simulink model "TorqueControlConfig"  (R2023b)
settings: Solver=VariableStepAuto  StartTime=0.0  StopTime=20  RelTol=1e-3
PostLoadFcn:
  | run('ParametricRobotLoader.m')
  | run('ParametricRobotParameters');
  | TsCtrl=0.005
  | Config.Mode=ones(1,6)
  | Config.Value = zeros(1,6)
undefined symbols (not defined in the file): ctrlLowerLimit, ctrlUpperLimit
libraries: nesl_utility x19, fl_lib x6, slpidlib x6, sm_lib x3, simulink x2, robotmaniplib x1
(part 1 of 2)
settings Model: PauseTimes=1  Creator=jjha  LastModifiedBy=abirdas
settings OptimizationCC: ReuseModelBlockBuffer=off
settings SimscapeCC: SimscapeLogType=all

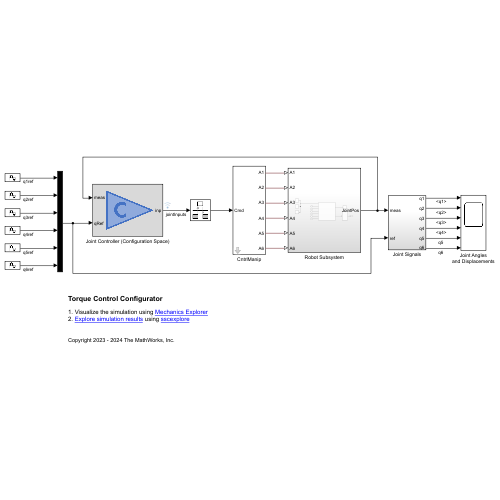
[thumbnail: Simulink's stored preview of the top-level diagram]
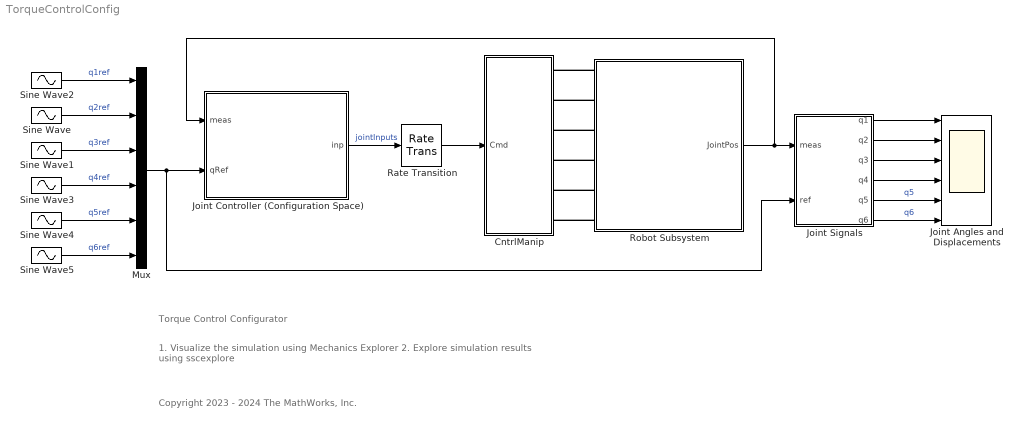
== system TorqueControlConfig ==
  note: Torque Control Configurator
  note: 1. Visualize the simulation using Mechanics Explorer
      | 2. Explore simulation results using sscexplore
  note: Copyright 2023 - 2024 The MathWorks, Inc.
  CntrlManip : Subsystem  mask{ControlSel=[1,1,1,1,1,1], ControlVal=Config.Value}
      mask prompts: ControlSel "Control Manipulator Selector"; ControlVal "Control Manipulator Value"
  Joint Angles and Displacements : Scope  NumInputPorts=6
  Joint Controller (Configuration Space) : Subsystem  VariantControl=ctrlType==1
      mask Display: image('Controller.PNG')
  Joint Signals : Subsystem
  Mux : Mux  Inputs=6
  Rate Transition : RateTransition
  Robot Subsystem : Subsystem
  Sine Wave : Sin  Amplitude=pi/4  Frequency=2  SampleTime=TsCtrl
  Sine Wave1 : Sin  Amplitude=pi/2  Frequency=1.5  SampleTime=TsCtrl
  Sine Wave2 : Sin  Amplitude=2*pi/3  Frequency=0.4  SampleTime=TsCtrl
  Sine Wave3 : Sin  Amplitude=pi/3  SampleTime=TsCtrl
  Sine Wave4 : Sin  Amplitude=2  Frequency=0.5  SampleTime=TsCtrl
  Sine Wave5 : Sin  Amplitude=pi/3  Frequency=2  SampleTime=TsCtrl
  wires:
  Joint Signals/4(q4) -> Joint Angles and Displacements/4
  Joint Signals/2(q2) -> Joint Angles and Displacements/2
  Robot Subsystem/1(JointPos) -> Joint Controller (Configuration Space)/1(meas), Joint Signals/1(meas)
  Joint Signals/3(q3) -> Joint Angles and Displacements/3
  Joint Signals/1(q1) -> Joint Angles and Displacements/1
  Joint Controller (Configuration Space)/1(inp) -> Rate Transition/1  "jointInputs"
  Mux/1 -> Joint Signals/2(ref), Joint Controller (Configuration Space)/2(qRef)
  Joint Signals/5(q5) -> Joint Angles and Displacements/5  "q5"
  Joint Signals/6(q6) -> Joint Angles and Displacements/6  "q6"
  Sine Wave2/1 -> Mux/1  "q1ref"
  Sine Wave/1 -> Mux/2  "q2ref"
  Sine Wave1/1 -> Mux/3  "q3ref"
  Sine Wave3/1 -> Mux/4  "q4ref"
  Sine Wave4/1 -> Mux/5  "q5ref"
  Sine Wave5/1 -> Mux/6  "q6ref"
  Rate Transition/1 -> CntrlManip/1(Cmd)
  connections:
  Robot Subsystem/LConn1 -- CntrlManip/RConn1
  Robot Subsystem/LConn2 -- CntrlManip/RConn2
  Robot Subsystem/LConn3 -- CntrlManip/RConn3
  Robot Subsystem/LConn4 -- CntrlManip/RConn4
  Robot Subsystem/LConn5 -- CntrlManip/RConn5
  Robot Subsystem/LConn6 -- CntrlManip/RConn6

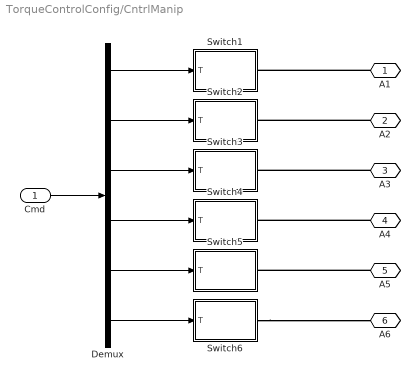
== system TorqueControlConfig/CntrlManip ==
  Cmd : Inport
  Demux : Demux  Outputs=6
  Switch1 : Subsystem  mask{ManipCtrl=ControlSel(1), ManipValue=ControlVal(1)}
      mask prompts: ManipCtrl "Control Selector"; ManipValue "Control Value"
      mask DialogControl Manipulator Prompt: Torque or Motion control
  Switch2 : Subsystem  mask{ManipCtrl=ControlSel(2), ManipValue=ControlVal(2)}
      mask prompts: ManipCtrl "Control Selector"; ManipValue "Control Value"
      mask DialogControl Manipulator Prompt: Torque or Motion control
  Switch3 : Subsystem  mask{ManipCtrl=ControlSel(3), ManipValue=ControlVal(3)}
      mask prompts: ManipCtrl "Control Selector"; ManipValue "Control Value"
      mask DialogControl Manipulator Prompt: Torque or Motion control
  Switch4 : Subsystem  mask{ManipCtrl=ControlSel(4), ManipValue=ControlVal(4)}
      mask prompts: ManipCtrl "Control Selector"; ManipValue "Control Value"
      mask DialogControl Manipulator Prompt: Torque or Motion control
  Switch5 : Subsystem  mask{ManipCtrl=ControlSel(5), ManipValue=ControlVal(5)}
      mask prompts: ManipCtrl "Control Selector"; ManipValue "Control Value"
      mask DialogControl Manipulator Prompt: Torque or Motion control
  Switch6 : Subsystem  mask{ManipCtrl=ControlSel(6), ManipValue=ControlVal(6)}
      mask prompts: ManipCtrl "Control Selector"; ManipValue "Control Value"
      mask DialogControl Manipulator Prompt: Torque or Motion control
  A1 : PMIOPort  Side=Right
  A2 : PMIOPort  Port=2  Side=Right
  A3 : PMIOPort  Port=3  Side=Right
  A4 : PMIOPort  Port=4  Side=Right
  A5 : PMIOPort  Port=5  Side=Right
  A6 : PMIOPort  Port=6  Side=Right
  wires:
  Cmd/1 -> Demux/1
  Demux/1 -> Switch1/1(T)
  Demux/2 -> Switch2/1(T)
  Demux/3 -> Switch3/1(T)
  Demux/4 -> Switch4/1(T)
  Demux/5 -> Switch5/1(T)
  Demux/6 -> Switch6/1(T)
  connections:
  A1/RConn1 -- Switch1/RConn1
  A2/RConn1 -- Switch2/RConn1
  A3/RConn1 -- Switch3/RConn1
  A4/RConn1 -- Switch4/RConn1
  A5/RConn1 -- Switch5/RConn1
  Switch6/RConn1 -- A6/RConn1

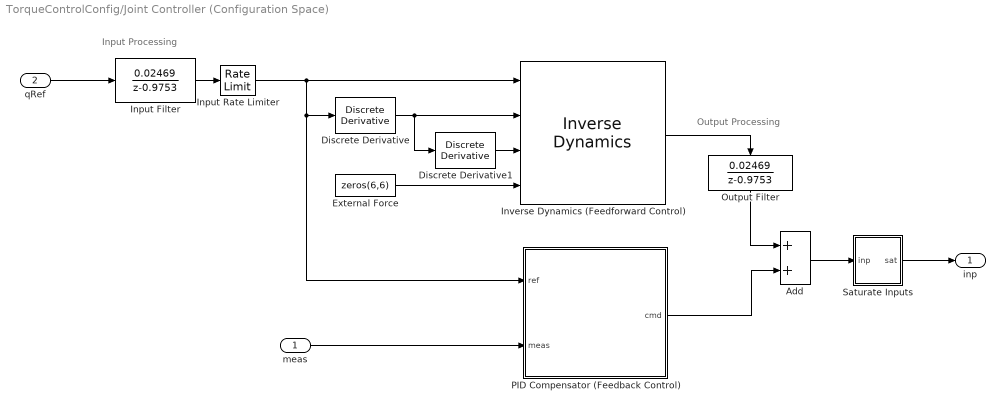
== system TorqueControlConfig/Joint Controller (Configuration Space) ==
  note: Input Processing
  note: Output Processing
  meas : Inport  SampleTime=TsCtrl
  qRef : Inport  Port=2  SampleTime=TsCtrl
  Add : Sum
  Discrete Derivative : simulink/Discrete/Discrete Derivative  gainval=1.0  ICPrevScaledInput=0.0  OutMin=[]  OutMax=[]  OutDataType=fixdt(1, 16)  OutScaling=2^-10  DoSatur=off
  Discrete Derivative1 : simulink/Discrete/Discrete Derivative  gainval=1.0  ICPrevScaledInput=0.0  OutMin=[]  OutMax=[]  OutDataType=fixdt(1, 16)  OutScaling=2^-10  DoSatur=off
  External Force : Constant  Value=zeros(6,6)
  Input Rate Limiter : RateLimiter  RisingSlewLimit=pi  FallingSlewLimit=-pi  SampleTimeMode=inherited
  Input Filter : DiscreteTransferFcn  Numerator=0.02469  Denominator=[1 -0.9753]
  Inverse Dynamics (Feedforward Control) : robotmaniplib/Inverse Dynamics  RigidBodyTree=robotParametric  SimulateUsing=Interpreted execution
  Output Filter : DiscreteTransferFcn  Numerator=0.02469  Denominator=[1 -0.9753]
  PID Compensator (Feedback Control) : Subsystem
  Saturate Inputs : Subsystem
  inp : Outport  SampleTime=TsCtrl  VectorParamsAs1DForOutWhenUnconnected=off
  wires:
  Add/1 -> Saturate Inputs/1(inp)
  Inverse Dynamics (Feedforward Control)/1 -> Output Filter/1
  meas/1 -> PID Compensator (Feedback Control)/2(meas)
  Discrete Derivative1/1 -> Inverse Dynamics (Feedforward Control)/3
  Input Rate Limiter/1 -> PID Compensator (Feedback Control)/1(ref), Discrete Derivative/1, Inverse Dynamics (Feedforward Control)/1
  Discrete Derivative/1 -> Discrete Derivative1/1, Inverse Dynamics (Feedforward Control)/2
  External Force/1 -> Inverse Dynamics (Feedforward Control)/4
  qRef/1 -> Input Filter/1
  Input Filter/1 -> Input Rate Limiter/1
  Output Filter/1 -> Add/1
  PID Compensator (Feedback Control)/1(cmd) -> Add/2
  Saturate Inputs/1(sat) -> inp/1

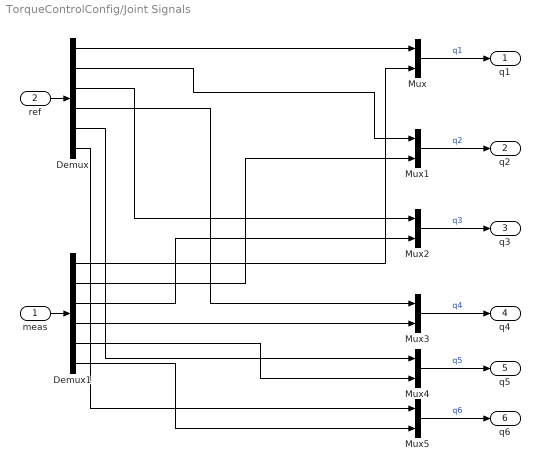
== system TorqueControlConfig/Joint Signals ==
  meas : Inport
  ref : Inport  Port=2
  Demux : Demux  Outputs=6
  Demux1 : Demux  Outputs=6
  Mux{,1..5} (6 alike) : Mux  Inputs=2
  q1 : Outport  VectorParamsAs1DForOutWhenUnconnected=off
  q2 : Outport  Port=2  VectorParamsAs1DForOutWhenUnconnected=off
  q3 : Outport  Port=3  VectorParamsAs1DForOutWhenUnconnected=off
  q4 : Outport  Port=4  VectorParamsAs1DForOutWhenUnconnected=off
  q5 : Outport  Port=5  VectorParamsAs1DForOutWhenUnconnected=off
  q6 : Outport  Port=6  VectorParamsAs1DForOutWhenUnconnected=off
  wires:
  Mux2/1 -> q3/1  "q3"
  ref/1 -> Demux/1
  Mux3/1 -> q4/1  "q4"
  Mux/1 -> q1/1  "q1"
  meas/1 -> Demux1/1
  Demux/1 -> Mux/1
  Demux1/1 -> Mux/2
  Mux1/1 -> q2/1  "q2"
  Demux/2 -> Mux1/1
  Demux1/2 -> Mux1/2
  Demux/3 -> Mux2/1
  Demux1/3 -> Mux2/2
  Demux1/4 -> Mux3/2
  Demux/4 -> Mux3/1
  Demux/5 -> Mux4/1
  Demux1/5 -> Mux4/2
  Mux4/1 -> q5/1  "q5"
  Demux/6 -> Mux5/1
  Demux1/6 -> Mux5/2
  Mux5/1 -> q6/1  "q6"

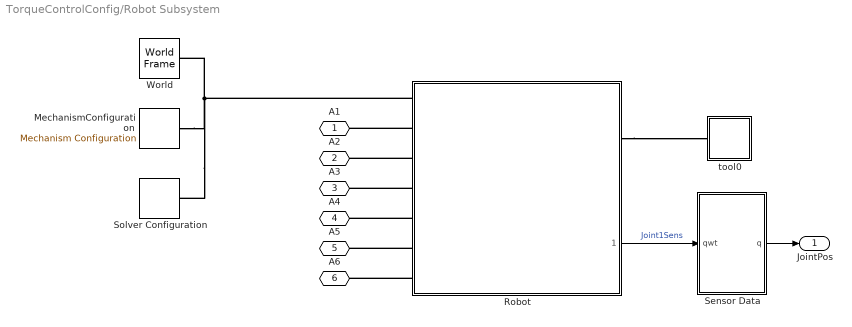
== system TorqueControlConfig/Robot Subsystem ==
  " Robot" : Subsystem  ReferencedSubsystem=ParametricRobotSubsystem  workflow=[1,1,1,1,1,1]
      settings: PortSchema="{\"entries\":[{\"content\":{\"sides\":[{\"content\":{\"connectorIds\":[\"LConn1\",\"LConn2\",\"LConn3\",\"LConn4\",\"LConn5\",\"LConn6\",\"LConn7\"]},\"type\":\"ConnectorPlacement.EquallySpacedRectSide\",\"uuid\":\"c330c7ea-b696-48e5-82ba-07054b6b44ca\"},{\"content\":{\"connectorIds\":[\"RConn1\",\"Out1\"],\"side\":\"RIGHT\"},\"type\":\"ConnectorPlacement.EquallySpacedRectSide\",\"uuid\":\"07fee86c-e3ee-4c7c-b794-151204654c18\"},{\"content\":{\"side\":\"TOP\"},\"type\":\"ConnectorPlacement.EquallySpacedRectSide\",\"uuid\":\"0a64827e-1227-40a0-b694-a7747fcb62b0\"}]},\"type\":\"ConnectorPlacement.EquallySpacedConnector\",\"uuid\":\"7ecd90c7-a601-4571-92be-f9b4e263de3c\"}],\"packageUris\":[\"http://schema.mathworks.com/mf0/Connector/R2020b\"],\"version\":\"1.0\"}"
  MechanismConfiguration : sm_lib/Utilities/Mechanism Configuration  UniformGravity=Constant  GravityVector=[0 0 -9.80665]  GravityVectorUnits=m/s^2  LinearizationDelta=0.001  JointModeTransitionNonlinearIterations=2
  Sensor Data : Subsystem
  Solver Configuration : nesl_utility/Solver Configuration  PhysicalDomain=network_engine_domain  SubClassName=solver  LeftPortType=input  RightPortType=generic  Tones=[]  Harmonics=[]  SimulateNoise=off  Profile=off  UseLocalSampling=off  EnableSwitchedLinearOptims=on  FrequencyDomain=off  UseCCode=off  RelTol=0.001  AbsTol=0.001  MinStep=1e-09  ToWorkspace=off  RevertToSquareIcSolve=off  NumHomotopyIterations=100  PhasorMode=off  PhasorModeNumHarmonics=1  ConsistencySolver=NEWTON_XTOL_AFTER_FTOL  IndexReductionMethod=DerivativeReplacement  DoDC=off  ResidualTolerance=1e-09  ConsistencyTolSource=GLOBAL  ConsistencyAbsTol=0.001  ConsistencyRelTol=0.001  ConsistencyTolFactor=0.001  UseLocalSolver=off  LocalSolverChoice=NE_BACKWARD_EULER_ADVANCER  ResolveIndetEquations=on  FunctionEvalNumThread=1  LocalSolverSampleTime=0.01  DoFixedCost=off  MaxNonlinIter=3  MaxModeIter=2  ComputeImpulses=off  ImpulseIterations=2  LinearAlgebra=auto  LinearAlgebraNumThread=0  EquationFormulation=NE_TIME_EF  DelaysMemoryBudget=1024  AutomaticFiltering=on  FilteringTimeConstant=0.001  PartitionStorageMethod=AS_NEEDED  PartitionMemoryBudget=1024  PartitionMethod=ROBUST  MultibodyUseLocalSolver=off  MultibodyLocalSolverChoice=ODE1  MultibodyLocalSolverSampleTime=0.001
  World : sm_lib/Frames and Transforms/World Frame
  tool0 : Subsystem
  A1 : PMIOPort  Side=Left
  A2 : PMIOPort  Port=2  Side=Left
  A3 : PMIOPort  Port=3  Side=Left
  A4 : PMIOPort  Port=4  Side=Left
  A5 : PMIOPort  Port=5  Side=Left
  A6 : PMIOPort  Port=6  Side=Left
  JointPos : Outport  VectorParamsAs1DForOutWhenUnconnected=off
  wires:
  Sensor Data/1(q) -> JointPos/1
  " Robot"/1 -> Sensor Data/1(qwt)  "Joint1Sens"
  connections:
  " Robot"/LConn1 -- World/RConn1 -- Solver Configuration/RConn1 -- MechanismConfiguration/RConn1
  " Robot"/LConn3 -- A2/RConn1
  " Robot"/LConn5 -- A4/RConn1
  " Robot"/LConn6 -- A5/RConn1
  " Robot"/LConn7 -- A6/RConn1
  " Robot"/LConn4 -- A3/RConn1
  " Robot"/RConn1 -- tool0/LConn1
  " Robot"/LConn2 -- A1/RConn1

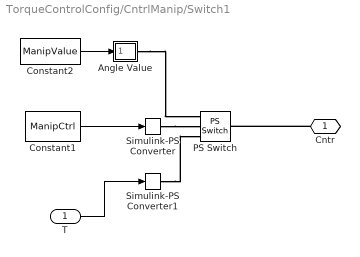
== system TorqueControlConfig/CntrlManip/Switch1 ==
  T : Inport
  Angle Value : Subsystem
  Constant1 : Constant  Value=ManipCtrl
  Constant2 : Constant  Value=ManipValue
  PS Switch : fl_lib/Physical Signals/Nonlinear Operators/PS Switch  Threshold=1.5
      settings: InternalSimscapePortConfiguration="{\"Bottom\":[],\"Left\":[{\"id\":\"I1\",\"label\":\"\",\"type\":\"input\"},{\"id\":\"I2\",\"label\":\"\",\"type\":\"input\"},{\"id\":\"I3\",\"label\":\"\",\"type\":\"input\"}],\"Right\":[{\"id\":\"O\",\"label\":\"\",\"type\":\"output\"}],\"Top\":[]}"
  Simulink-PS Converter : nesl_utility/Simulink-PS Converter  PhysicalDomain=network_engine_domain  SubClassName=ps_input  LeftPortType=input  RightPortType=output  PseudoPeriodic=off  Frequencies=[]  NoiseDistribution=none  NoiseParameters=[]  Unit=1  AffineConversion=off  FilteringAndDerivatives=provide  SimscapeFilterOrder=1  InputFilterTimeConstant=0.001  UdotUserProvided=0
  Simulink-PS Converter1 : nesl_utility/Simulink-PS Converter  PhysicalDomain=network_engine_domain  SubClassName=ps_input  LeftPortType=input  RightPortType=output  PseudoPeriodic=off  Frequencies=[]  NoiseDistribution=none  NoiseParameters=[]  Unit=1  AffineConversion=off  FilteringAndDerivatives=provide  SimscapeFilterOrder=1  InputFilterTimeConstant=0.001  UdotUserProvided=0
  Cntr : PMIOPort  Side=Right
  wires:
  T/1 -> Simulink-PS Converter1/1
  Constant1/1 -> Simulink-PS Converter/1
  Constant2/1 -> Angle Value/1(" ")
  connections:
  Angle Value/RConn1 -- PS Switch/LConn1
  Simulink-PS Converter/RConn1 -- PS Switch/LConn2
  Simulink-PS Converter1/RConn1 -- PS Switch/LConn3
  Cntr/RConn1 -- PS Switch/RConn1

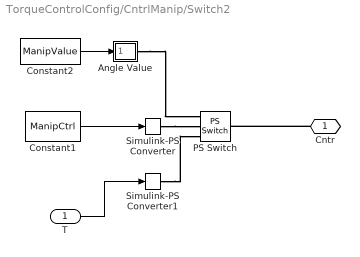
== system TorqueControlConfig/CntrlManip/Switch2 ==
  T : Inport
  Angle Value : Subsystem
  Constant1 : Constant  Value=ManipCtrl
  Constant2 : Constant  Value=ManipValue
  PS Switch : fl_lib/Physical Signals/Nonlinear Operators/PS Switch  Threshold=1.5
      settings: InternalSimscapePortConfiguration="{\"Bottom\":[],\"Left\":[{\"id\":\"I1\",\"label\":\"\",\"type\":\"input\"},{\"id\":\"I2\",\"label\":\"\",\"type\":\"input\"},{\"id\":\"I3\",\"label\":\"\",\"type\":\"input\"}],\"Right\":[{\"id\":\"O\",\"label\":\"\",\"type\":\"output\"}],\"Top\":[]}"
  Simulink-PS Converter : nesl_utility/Simulink-PS Converter  PhysicalDomain=network_engine_domain  SubClassName=ps_input  LeftPortType=input  RightPortType=output  PseudoPeriodic=off  Frequencies=[]  NoiseDistribution=none  NoiseParameters=[]  Unit=1  AffineConversion=off  FilteringAndDerivatives=provide  SimscapeFilterOrder=1  InputFilterTimeConstant=0.001  UdotUserProvided=0
  Simulink-PS Converter1 : nesl_utility/Simulink-PS Converter  PhysicalDomain=network_engine_domain  SubClassName=ps_input  LeftPortType=input  RightPortType=output  PseudoPeriodic=off  Frequencies=[]  NoiseDistribution=none  NoiseParameters=[]  Unit=1  AffineConversion=off  FilteringAndDerivatives=provide  SimscapeFilterOrder=1  InputFilterTimeConstant=0.001  UdotUserProvided=0
  Cntr : PMIOPort  Side=Right
  wires:
  Constant2/1 -> Angle Value/1(" ")
  Constant1/1 -> Simulink-PS Converter/1
  T/1 -> Simulink-PS Converter1/1
  connections:
  Cntr/RConn1 -- PS Switch/RConn1
  Simulink-PS Converter1/RConn1 -- PS Switch/LConn3
  Simulink-PS Converter/RConn1 -- PS Switch/LConn2
  Angle Value/RConn1 -- PS Switch/LConn1

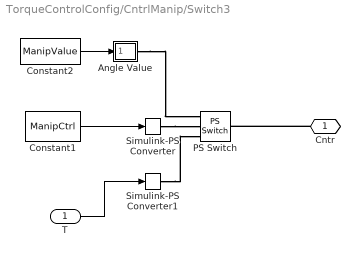
== system TorqueControlConfig/CntrlManip/Switch3 ==
  T : Inport
  Angle Value : Subsystem
  Constant1 : Constant  Value=ManipCtrl
  Constant2 : Constant  Value=ManipValue
  PS Switch : fl_lib/Physical Signals/Nonlinear Operators/PS Switch  Threshold=1.5
      settings: InternalSimscapePortConfiguration="{\"Bottom\":[],\"Left\":[{\"id\":\"I1\",\"label\":\"\",\"type\":\"input\"},{\"id\":\"I2\",\"label\":\"\",\"type\":\"input\"},{\"id\":\"I3\",\"label\":\"\",\"type\":\"input\"}],\"Right\":[{\"id\":\"O\",\"label\":\"\",\"type\":\"output\"}],\"Top\":[]}"
  Simulink-PS Converter : nesl_utility/Simulink-PS Converter  PhysicalDomain=network_engine_domain  SubClassName=ps_input  LeftPortType=input  RightPortType=output  PseudoPeriodic=off  Frequencies=[]  NoiseDistribution=none  NoiseParameters=[]  Unit=1  AffineConversion=off  FilteringAndDerivatives=provide  SimscapeFilterOrder=1  InputFilterTimeConstant=0.001  UdotUserProvided=0
  Simulink-PS Converter1 : nesl_utility/Simulink-PS Converter  PhysicalDomain=network_engine_domain  SubClassName=ps_input  LeftPortType=input  RightPortType=output  PseudoPeriodic=off  Frequencies=[]  NoiseDistribution=none  NoiseParameters=[]  Unit=1  AffineConversion=off  FilteringAndDerivatives=provide  SimscapeFilterOrder=1  InputFilterTimeConstant=0.001  UdotUserProvided=0
  Cntr : PMIOPort  Side=Right
  wires:
  T/1 -> Simulink-PS Converter1/1
  Constant1/1 -> Simulink-PS Converter/1
  Constant2/1 -> Angle Value/1(" ")
  connections:
  Angle Value/RConn1 -- PS Switch/LConn1
  Simulink-PS Converter/RConn1 -- PS Switch/LConn2
  Simulink-PS Converter1/RConn1 -- PS Switch/LConn3
  Cntr/RConn1 -- PS Switch/RConn1

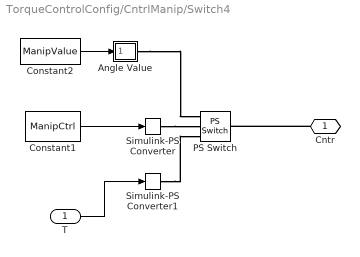
== system TorqueControlConfig/CntrlManip/Switch4 ==
  T : Inport
  Angle Value : Subsystem
  Constant1 : Constant  Value=ManipCtrl
  Constant2 : Constant  Value=ManipValue
  PS Switch : fl_lib/Physical Signals/Nonlinear Operators/PS Switch  Threshold=1.5
      settings: InternalSimscapePortConfiguration="{\"Bottom\":[],\"Left\":[{\"id\":\"I1\",\"label\":\"\",\"type\":\"input\"},{\"id\":\"I2\",\"label\":\"\",\"type\":\"input\"},{\"id\":\"I3\",\"label\":\"\",\"type\":\"input\"}],\"Right\":[{\"id\":\"O\",\"label\":\"\",\"type\":\"output\"}],\"Top\":[]}"
  Simulink-PS Converter : nesl_utility/Simulink-PS Converter  PhysicalDomain=network_engine_domain  SubClassName=ps_input  LeftPortType=input  RightPortType=output  PseudoPeriodic=off  Frequencies=[]  NoiseDistribution=none  NoiseParameters=[]  Unit=1  AffineConversion=off  FilteringAndDerivatives=provide  SimscapeFilterOrder=1  InputFilterTimeConstant=0.001  UdotUserProvided=0
  Simulink-PS Converter1 : nesl_utility/Simulink-PS Converter  PhysicalDomain=network_engine_domain  SubClassName=ps_input  LeftPortType=input  RightPortType=output  PseudoPeriodic=off  Frequencies=[]  NoiseDistribution=none  NoiseParameters=[]  Unit=1  AffineConversion=off  FilteringAndDerivatives=provide  SimscapeFilterOrder=1  InputFilterTimeConstant=0.001  UdotUserProvided=0
  Cntr : PMIOPort  Side=Right
  wires:
  Constant2/1 -> Angle Value/1(" ")
  Constant1/1 -> Simulink-PS Converter/1
  T/1 -> Simulink-PS Converter1/1
  connections:
  Cntr/RConn1 -- PS Switch/RConn1
  Simulink-PS Converter1/RConn1 -- PS Switch/LConn3
  Simulink-PS Converter/RConn1 -- PS Switch/LConn2
  Angle Value/RConn1 -- PS Switch/LConn1

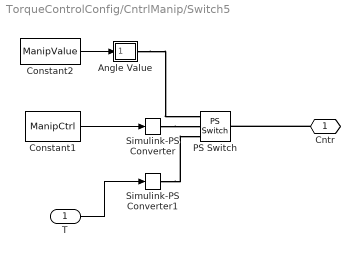
== system TorqueControlConfig/CntrlManip/Switch5 ==
  T : Inport
  Angle Value : Subsystem
  Constant1 : Constant  Value=ManipCtrl
  Constant2 : Constant  Value=ManipValue
  PS Switch : fl_lib/Physical Signals/Nonlinear Operators/PS Switch  Threshold=1.5
      settings: InternalSimscapePortConfiguration="{\"Bottom\":[],\"Left\":[{\"id\":\"I1\",\"label\":\"\",\"type\":\"input\"},{\"id\":\"I2\",\"label\":\"\",\"type\":\"input\"},{\"id\":\"I3\",\"label\":\"\",\"type\":\"input\"}],\"Right\":[{\"id\":\"O\",\"label\":\"\",\"type\":\"output\"}],\"Top\":[]}"
  Simulink-PS Converter : nesl_utility/Simulink-PS Converter  PhysicalDomain=network_engine_domain  SubClassName=ps_input  LeftPortType=input  RightPortType=output  PseudoPeriodic=off  Frequencies=[]  NoiseDistribution=none  NoiseParameters=[]  Unit=1  AffineConversion=off  FilteringAndDerivatives=provide  SimscapeFilterOrder=1  InputFilterTimeConstant=0.001  UdotUserProvided=0
  Simulink-PS Converter1 : nesl_utility/Simulink-PS Converter  PhysicalDomain=network_engine_domain  SubClassName=ps_input  LeftPortType=input  RightPortType=output  PseudoPeriodic=off  Frequencies=[]  NoiseDistribution=none  NoiseParameters=[]  Unit=1  AffineConversion=off  FilteringAndDerivatives=provide  SimscapeFilterOrder=1  InputFilterTimeConstant=0.001  UdotUserProvided=0
  Cntr : PMIOPort  Side=Right
  wires:
  T/1 -> Simulink-PS Converter1/1
  Constant1/1 -> Simulink-PS Converter/1
  Constant2/1 -> Angle Value/1(" ")
  connections:
  Angle Value/RConn1 -- PS Switch/LConn1
  Simulink-PS Converter/RConn1 -- PS Switch/LConn2
  Simulink-PS Converter1/RConn1 -- PS Switch/LConn3
  Cntr/RConn1 -- PS Switch/RConn1

== system TorqueControlConfig/CntrlManip/Switch6 ==
  T : Inport
  Angle Value : Subsystem
  Constant1 : Constant  Value=ManipCtrl
  Constant2 : Constant  Value=ManipValue
  PS Switch : fl_lib/Physical Signals/Nonlinear Operators/PS Switch  Threshold=1.5
      settings: InternalSimscapePortConfiguration="{\"Bottom\":[],\"Left\":[{\"id\":\"I1\",\"label\":\"\",\"type\":\"input\"},{\"id\":\"I2\",\"label\":\"\",\"type\":\"input\"},{\"id\":\"I3\",\"label\":\"\",\"type\":\"input\"}],\"Right\":[{\"id\":\"O\",\"label\":\"\",\"type\":\"output\"}],\"Top\":[]}"
  Simulink-PS Converter : nesl_utility/Simulink-PS Converter  PhysicalDomain=network_engine_domain  SubClassName=ps_input  LeftPortType=input  RightPortType=output  PseudoPeriodic=off  Frequencies=[]  NoiseDistribution=none  NoiseParameters=[]  Unit=1  AffineConversion=off  FilteringAndDerivatives=provide  SimscapeFilterOrder=1  InputFilterTimeConstant=0.001  UdotUserProvided=0
  Simulink-PS Converter1 : nesl_utility/Simulink-PS Converter  PhysicalDomain=network_engine_domain  SubClassName=ps_input  LeftPortType=input  RightPortType=output  PseudoPeriodic=off  Frequencies=[]  NoiseDistribution=none  NoiseParameters=[]  Unit=1  AffineConversion=off  FilteringAndDerivatives=provide  SimscapeFilterOrder=1  InputFilterTimeConstant=0.001  UdotUserProvided=0
  Cntr : PMIOPort  Side=Right
  wires:
  Constant2/1 -> Angle Value/1(" ")
  Constant1/1 -> Simulink-PS Converter/1
  T/1 -> Simulink-PS Converter1/1
  connections:
  Cntr/RConn1 -- PS Switch/RConn1
  Simulink-PS Converter1/RConn1 -- PS Switch/LConn3
  Simulink-PS Converter/RConn1 -- PS Switch/LConn2
  Angle Value/RConn1 -- PS Switch/LConn1

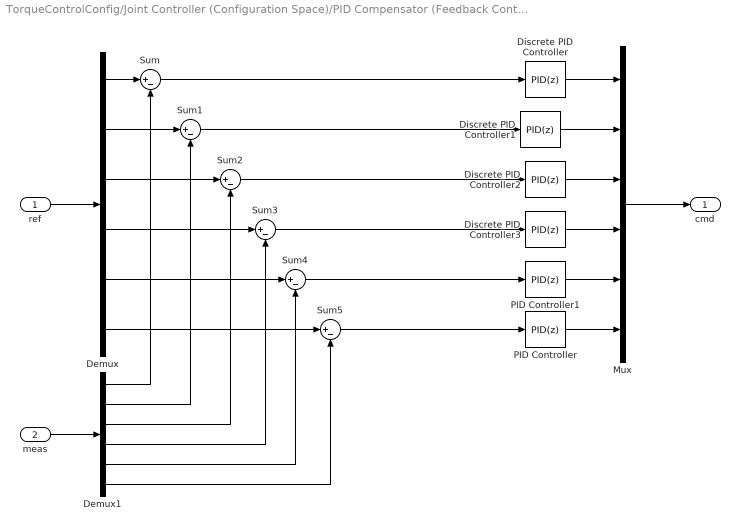
== system TorqueControlConfig/Joint Controller (Configuration Space)/PID Compensator (Feedback Control) ==
  ref : Inport
  meas : Inport  Port=2
  Demux : Demux  Outputs=6
  Demux1 : Demux  Outputs=6
  Discrete PID Controller : slpidlib/PID Controller  Controller=PID  Form=Parallel  TimeDomain=Discrete-time  UseExternalTs=off  SampleTime=-1  IntegratorMethod=Forward Euler  FilterMethod=Forward Euler  ControllerParametersSource=internal  P=3  I=0.305808289397669  UseKiTs=off  D=3.38874529476647  N=100  UseFilter=on  TunerSelectOption=Transfer Function Based (PID Tuner App)  InitialConditionSource=internal  InitialConditionForIntegrator=0  InitialConditionForFilter=0  DifferentiatorICPrevScaledInput=0  ExternalReset=none  TrackingMode=off  Kt=1  LimitOutput=off  SatLimitsSource=internal  UpperSaturationLimit=ctrlUpperLimit  LowerSaturationLimit=ctrlLowerLimit  LinearizeAsGain=off  AntiWindupMode=clamping  Kb=1  LimitIntegrator=off  UpperIntegratorSaturationLimit=inf  LowerIntegratorSaturationLimit=-inf  POutMin=[]  POutMax=[]  IOutMin=[]  IOutMax=[]  DOutMin=[]  DOutMax=[]  NOutMin=[]  NOutMax=[]  SumOutMin=[]  SumOutMax=[]  SaturationOutMin=[]  SaturationOutMax=[]  PParamMin=[]  PParamMax=[]  IParamMin=[]  IParamMax=[]  DParamMin=[]  DParamMax=[]  NParamMin=[]  NParamMax=[]  KbParamMin=[]  KbParamMax=[]  KtParamMin=[]  KtParamMax=[]  KbOutMin=[]  KbOutMax=[]  KtOutMin=[]  KtOutMax=[]  IntegratorOutMin=[]  IntegratorOutMax=[]  FilterOutMin=[]  FilterOutMax=[]  SumI1OutMin=[]  SumI1OutMax=[]  SumI2OutMin=[]  SumI2OutMax=[]  SumI3OutMin=[]  SumI3OutMax=[]  SumI4OutMin=[]  SumI4OutMax=[]  SumDOutMin=[]  SumDOutMax=[]  DifferentiatorOutMin=[]  DifferentiatorOutMax=[]  FilterDiffOutCoefMin=[]  FilterDiffOutCoefMax=[]  ReciprocalOutMin=[]  ReciprocalOutMax=[]  SumDenOutMin=[]  SumDenOutMax=[]  SumNumOutMin=[]  SumNumOutMax=[]  DivideOutMin=[]  DivideOutMax=[]  UdiffTsProdOutMin=[]  UdiffTsProdOutMax=[]  NTsProdOutMin=[]  NTsProdOutMax=[]  UintegralTsProdOutMin=[]  UintegralTsProdOutMax=[]  UngainTsProdOutMin=[]  UngainTsProdOutMax=[]  ClampingZeroOutDataTypeStr=Inherit: Inherit via back propagation  ClampingZeroOutMin=[]  ClampingZeroOutMax=[]  FilterDenConstantOutDataTypeStr=Inherit: Inherit via back propagation  FilterDenConstantOutMin=[]  FilterDenConstantOutMax=[]  PCopyOutDataTypeStr=Inherit: Inherit via back propagation  PCopyOutMin=[]  PCopyOutMax=[]  NCopyOutDataTypeStr=Inherit: Inherit via back propagation  NCopyOutMin=[]  NCopyOutMax=[]  IntegratorContinuousStateAttributes=''  IntegratorStateMustResolveToSignalObject=off  IntegratorRTWStateStorageClass=Auto  FilterContinuousStateAttributes=''  FilterStateMustResolveToSignalObject=off  FilterRTWStateStorageClass=Auto  ParallelPVariant=InternalParameters  IdealPVariant=Disabled  IVariant=InternalParameters  DVariant=InternalParameters  IntegratorVariant=Discrete  SatVariant=Disabled  AWVariant=Passthrough  PCopyVariant=Disabled  TRVariant=Disabled  FdbkBlocksVariant=Forward  IdealPFdbkVariant=Disabled  SatFdbkVariant=Disabled  DerivativeFilterVariant=ForwardEulerFilter  NVariant=InternalParameters  NCopyVariant=Disabled  FilterICVariant=InternalICsFilter  IntegratorICVariant=InternalICs  ExternalResetVariant=Disabled  TRSumVariant=Passthrough  SumFdbkVariant=Disabled  SumVariant=Sum_PID  TsampFilterVariant=InternalTs  TsampNgainVariant=Passthrough  TsampIntegralVariant=Disabled_SignalSpec  ExternalSaturationOutDataTypeStr=Inherit: Same as second input
  Discrete PID Controller1 : slpidlib/PID Controller  Controller=PID  Form=Parallel  TimeDomain=Discrete-time  UseExternalTs=off  SampleTime=-1  IntegratorMethod=Forward Euler  FilterMethod=Forward Euler  ControllerParametersSource=internal  P=110.696309330524  I=151.729850438955  UseKiTs=off  D=18.8321395774824  N=347.517442654489  UseFilter=on  TunerSelectOption=Transfer Function Based (PID Tuner App)  InitialConditionSource=internal  InitialConditionForIntegrator=0  InitialConditionForFilter=0  DifferentiatorICPrevScaledInput=0  ExternalReset=none  TrackingMode=off  Kt=1  LimitOutput=off  SatLimitsSource=internal  UpperSaturationLimit=ctrlUpperLimit  LowerSaturationLimit=ctrlLowerLimit  LinearizeAsGain=off  AntiWindupMode=clamping  Kb=1  LimitIntegrator=off  UpperIntegratorSaturationLimit=inf  LowerIntegratorSaturationLimit=-inf  POutMin=[]  POutMax=[]  IOutMin=[]  IOutMax=[]  DOutMin=[]  DOutMax=[]  NOutMin=[]  NOutMax=[]  SumOutMin=[]  SumOutMax=[]  SaturationOutMin=[]  SaturationOutMax=[]  PParamMin=[]  PParamMax=[]  IParamMin=[]  IParamMax=[]  DParamMin=[]  DParamMax=[]  NParamMin=[]  NParamMax=[]  KbParamMin=[]  KbParamMax=[]  KtParamMin=[]  KtParamMax=[]  KbOutMin=[]  KbOutMax=[]  KtOutMin=[]  KtOutMax=[]  IntegratorOutMin=[]  IntegratorOutMax=[]  FilterOutMin=[]  FilterOutMax=[]  SumI1OutMin=[]  SumI1OutMax=[]  SumI2OutMin=[]  SumI2OutMax=[]  SumI3OutMin=[]  SumI3OutMax=[]  SumI4OutMin=[]  SumI4OutMax=[]  SumDOutMin=[]  SumDOutMax=[]  DifferentiatorOutMin=[]  DifferentiatorOutMax=[]  FilterDiffOutCoefMin=[]  FilterDiffOutCoefMax=[]  ReciprocalOutMin=[]  ReciprocalOutMax=[]  SumDenOutMin=[]  SumDenOutMax=[]  SumNumOutMin=[]  SumNumOutMax=[]  DivideOutMin=[]  DivideOutMax=[]  UdiffTsProdOutMin=[]  UdiffTsProdOutMax=[]  NTsProdOutMin=[]  NTsProdOutMax=[]  UintegralTsProdOutMin=[]  UintegralTsProdOutMax=[]  UngainTsProdOutMin=[]  UngainTsProdOutMax=[]  ClampingZeroOutDataTypeStr=Inherit: Inherit via back propagation  ClampingZeroOutMin=[]  ClampingZeroOutMax=[]  FilterDenConstantOutDataTypeStr=Inherit: Inherit via back propagation  FilterDenConstantOutMin=[]  FilterDenConstantOutMax=[]  PCopyOutDataTypeStr=Inherit: Inherit via back propagation  PCopyOutMin=[]  PCopyOutMax=[]  NCopyOutDataTypeStr=Inherit: Inherit via back propagation  NCopyOutMin=[]  NCopyOutMax=[]  IntegratorContinuousStateAttributes=''  IntegratorStateMustResolveToSignalObject=off  IntegratorRTWStateStorageClass=Auto  FilterContinuousStateAttributes=''  FilterStateMustResolveToSignalObject=off  FilterRTWStateStorageClass=Auto  ParallelPVariant=InternalParameters  IdealPVariant=Disabled  IVariant=InternalParameters  DVariant=InternalParameters  IntegratorVariant=Discrete  SatVariant=Disabled  AWVariant=Passthrough  PCopyVariant=Disabled  TRVariant=Disabled  FdbkBlocksVariant=Forward  IdealPFdbkVariant=Disabled  SatFdbkVariant=Disabled  DerivativeFilterVariant=ForwardEulerFilter  NVariant=InternalParameters  NCopyVariant=Disabled  FilterICVariant=InternalICsFilter  IntegratorICVariant=InternalICs  ExternalResetVariant=Disabled  TRSumVariant=Passthrough  SumFdbkVariant=Disabled  SumVariant=Sum_PID  TsampFilterVariant=InternalTs  TsampNgainVariant=Passthrough  TsampIntegralVariant=Disabled_SignalSpec  ExternalSaturationOutDataTypeStr=Inherit: Same as second input
  Discrete PID Controller2 : slpidlib/PID Controller  Controller=PID  Form=Parallel  TimeDomain=Discrete-time  UseExternalTs=off  SampleTime=-1  IntegratorMethod=Forward Euler  FilterMethod=Forward Euler  ControllerParametersSource=internal  P=46.6071952200349  I=94.4566299090337  UseKiTs=off  D=5.35707582211615  N=102.069719279228  UseFilter=on  TunerSelectOption=Transfer Function Based (PID Tuner App)  InitialConditionSource=internal  InitialConditionForIntegrator=0  InitialConditionForFilter=0  DifferentiatorICPrevScaledInput=0  ExternalReset=none  TrackingMode=off  Kt=1  LimitOutput=off  SatLimitsSource=internal  UpperSaturationLimit=ctrlUpperLimit  LowerSaturationLimit=ctrlLowerLimit  LinearizeAsGain=off  AntiWindupMode=clamping  Kb=1  LimitIntegrator=off  UpperIntegratorSaturationLimit=inf  LowerIntegratorSaturationLimit=-inf  POutMin=[]  POutMax=[]  IOutMin=[]  IOutMax=[]  DOutMin=[]  DOutMax=[]  NOutMin=[]  NOutMax=[]  SumOutMin=[]  SumOutMax=[]  SaturationOutMin=[]  SaturationOutMax=[]  PParamMin=[]  PParamMax=[]  IParamMin=[]  IParamMax=[]  DParamMin=[]  DParamMax=[]  NParamMin=[]  NParamMax=[]  KbParamMin=[]  KbParamMax=[]  KtParamMin=[]  KtParamMax=[]  KbOutMin=[]  KbOutMax=[]  KtOutMin=[]  KtOutMax=[]  IntegratorOutMin=[]  IntegratorOutMax=[]  FilterOutMin=[]  FilterOutMax=[]  SumI1OutMin=[]  SumI1OutMax=[]  SumI2OutMin=[]  SumI2OutMax=[]  SumI3OutMin=[]  SumI3OutMax=[]  SumI4OutMin=[]  SumI4OutMax=[]  SumDOutMin=[]  SumDOutMax=[]  DifferentiatorOutMin=[]  DifferentiatorOutMax=[]  FilterDiffOutCoefMin=[]  FilterDiffOutCoefMax=[]  ReciprocalOutMin=[]  ReciprocalOutMax=[]  SumDenOutMin=[]  SumDenOutMax=[]  SumNumOutMin=[]  SumNumOutMax=[]  DivideOutMin=[]  DivideOutMax=[]  UdiffTsProdOutMin=[]  UdiffTsProdOutMax=[]  NTsProdOutMin=[]  NTsProdOutMax=[]  UintegralTsProdOutMin=[]  UintegralTsProdOutMax=[]  UngainTsProdOutMin=[]  UngainTsProdOutMax=[]  ClampingZeroOutDataTypeStr=Inherit: Inherit via back propagation  ClampingZeroOutMin=[]  ClampingZeroOutMax=[]  FilterDenConstantOutDataTypeStr=Inherit: Inherit via back propagation  FilterDenConstantOutMin=[]  FilterDenConstantOutMax=[]  PCopyOutDataTypeStr=Inherit: Inherit via back propagation  PCopyOutMin=[]  PCopyOutMax=[]  NCopyOutDataTypeStr=Inherit: Inherit via back propagation  NCopyOutMin=[]  NCopyOutMax=[]  IntegratorContinuousStateAttributes=''  IntegratorStateMustResolveToSignalObject=off  IntegratorRTWStateStorageClass=Auto  FilterContinuousStateAttributes=''  FilterStateMustResolveToSignalObject=off  FilterRTWStateStorageClass=Auto  ParallelPVariant=InternalParameters  IdealPVariant=Disabled  IVariant=InternalParameters  DVariant=InternalParameters  IntegratorVariant=Discrete  SatVariant=Disabled  AWVariant=Passthrough  PCopyVariant=Disabled  TRVariant=Disabled  FdbkBlocksVariant=Forward  IdealPFdbkVariant=Disabled  SatFdbkVariant=Disabled  DerivativeFilterVariant=ForwardEulerFilter  NVariant=InternalParameters  NCopyVariant=Disabled  FilterICVariant=InternalICsFilter  IntegratorICVariant=InternalICs  ExternalResetVariant=Disabled  TRSumVariant=Passthrough  SumFdbkVariant=Disabled  SumVariant=Sum_PID  TsampFilterVariant=InternalTs  TsampNgainVariant=Passthrough  TsampIntegralVariant=Disabled_SignalSpec  ExternalSaturationOutDataTypeStr=Inherit: Same as second input
  Discrete PID Controller3 : slpidlib/PID Controller  Controller=PID  Form=Parallel  TimeDomain=Discrete-time  UseExternalTs=off  SampleTime=-1  IntegratorMethod=Forward Euler  FilterMethod=Forward Euler  ControllerParametersSource=internal  P=3  I=0.2  UseKiTs=off  D=0.0831019668090638  N=338.744071172156  UseFilter=on  TunerSelectOption=Transfer Function Based (PID Tuner App)  InitialConditionSource=internal  InitialConditionForIntegrator=0  InitialConditionForFilter=0  DifferentiatorICPrevScaledInput=0  ExternalReset=none  TrackingMode=off  Kt=1  LimitOutput=off  SatLimitsSource=internal  UpperSaturationLimit=ctrlUpperLimit  LowerSaturationLimit=ctrlLowerLimit  LinearizeAsGain=off  AntiWindupMode=clamping  Kb=1  LimitIntegrator=off  UpperIntegratorSaturationLimit=inf  LowerIntegratorSaturationLimit=-inf  POutMin=[]  POutMax=[]  IOutMin=[]  IOutMax=[]  DOutMin=[]  DOutMax=[]  NOutMin=[]  NOutMax=[]  SumOutMin=[]  SumOutMax=[]  SaturationOutMin=[]  SaturationOutMax=[]  PParamMin=[]  PParamMax=[]  IParamMin=[]  IParamMax=[]  DParamMin=[]  DParamMax=[]  NParamMin=[]  NParamMax=[]  KbParamMin=[]  KbParamMax=[]  KtParamMin=[]  KtParamMax=[]  KbOutMin=[]  KbOutMax=[]  KtOutMin=[]  KtOutMax=[]  IntegratorOutMin=[]  IntegratorOutMax=[]  FilterOutMin=[]  FilterOutMax=[]  SumI1OutMin=[]  SumI1OutMax=[]  SumI2OutMin=[]  SumI2OutMax=[]  SumI3OutMin=[]  SumI3OutMax=[]  SumI4OutMin=[]  SumI4OutMax=[]  SumDOutMin=[]  SumDOutMax=[]  DifferentiatorOutMin=[]  DifferentiatorOutMax=[]  FilterDiffOutCoefMin=[]  FilterDiffOutCoefMax=[]  ReciprocalOutMin=[]  ReciprocalOutMax=[]  SumDenOutMin=[]  SumDenOutMax=[]  SumNumOutMin=[]  SumNumOutMax=[]  DivideOutMin=[]  DivideOutMax=[]  UdiffTsProdOutMin=[]  UdiffTsProdOutMax=[]  NTsProdOutMin=[]  NTsProdOutMax=[]  UintegralTsProdOutMin=[]  UintegralTsProdOutMax=[]  UngainTsProdOutMin=[]  UngainTsProdOutMax=[]  ClampingZeroOutDataTypeStr=Inherit: Inherit via back propagation  ClampingZeroOutMin=[]  ClampingZeroOutMax=[]  FilterDenConstantOutDataTypeStr=Inherit: Inherit via back propagation  FilterDenConstantOutMin=[]  FilterDenConstantOutMax=[]  PCopyOutDataTypeStr=Inherit: Inherit via back propagation  PCopyOutMin=[]  PCopyOutMax=[]  NCopyOutDataTypeStr=Inherit: Inherit via back propagation  NCopyOutMin=[]  NCopyOutMax=[]  IntegratorContinuousStateAttributes=''  IntegratorStateMustResolveToSignalObject=off  IntegratorRTWStateStorageClass=Auto  FilterContinuousStateAttributes=''  FilterStateMustResolveToSignalObject=off  FilterRTWStateStorageClass=Auto  ParallelPVariant=InternalParameters  IdealPVariant=Disabled  IVariant=InternalParameters  DVariant=InternalParameters  IntegratorVariant=Discrete  SatVariant=Disabled  AWVariant=Passthrough  PCopyVariant=Disabled  TRVariant=Disabled  FdbkBlocksVariant=Forward  IdealPFdbkVariant=Disabled  SatFdbkVariant=Disabled  DerivativeFilterVariant=ForwardEulerFilter  NVariant=InternalParameters  NCopyVariant=Disabled  FilterICVariant=InternalICsFilter  IntegratorICVariant=InternalICs  ExternalResetVariant=Disabled  TRSumVariant=Passthrough  SumFdbkVariant=Disabled  SumVariant=Sum_PID  TsampFilterVariant=InternalTs  TsampNgainVariant=Passthrough  TsampIntegralVariant=Disabled_SignalSpec  ExternalSaturationOutDataTypeStr=Inherit: Same as second input
  Mux : Mux  Inputs=6
  PID Controller : slpidlib/PID Controller  Controller=PID  Form=Parallel  TimeDomain=Discrete-time  UseExternalTs=off  SampleTime=-1  IntegratorMethod=Forward Euler  FilterMethod=Forward Euler  ControllerParametersSource=internal  P=0.70209665780819  I=0.573117882850985  UseKiTs=off  D=0.0764302604976139  N=292.50677796255  UseFilter=on  TunerSelectOption=Transfer Function Based (PID Tuner App)  InitialConditionSource=internal  InitialConditionForIntegrator=0  InitialConditionForFilter=0  DifferentiatorICPrevScaledInput=0  ExternalReset=none  TrackingMode=off  Kt=1  LimitOutput=off  SatLimitsSource=internal  UpperSaturationLimit=inf  LowerSaturationLimit=-inf  LinearizeAsGain=on  AntiWindupMode=none  Kb=1  LimitIntegrator=off  UpperIntegratorSaturationLimit=inf  LowerIntegratorSaturationLimit=-inf  POutMin=[]  POutMax=[]  IOutMin=[]  IOutMax=[]  DOutMin=[]  DOutMax=[]  NOutMin=[]  NOutMax=[]  SumOutMin=[]  SumOutMax=[]  SaturationOutMin=[]  SaturationOutMax=[]  PParamMin=[]  PParamMax=[]  IParamMin=[]  IParamMax=[]  DParamMin=[]  DParamMax=[]  NParamMin=[]  NParamMax=[]  KbParamMin=[]  KbParamMax=[]  KtParamMin=[]  KtParamMax=[]  KbOutMin=[]  KbOutMax=[]  KtOutMin=[]  KtOutMax=[]  IntegratorOutMin=[]  IntegratorOutMax=[]  FilterOutMin=[]  FilterOutMax=[]  SumI1OutMin=[]  SumI1OutMax=[]  SumI2OutMin=[]  SumI2OutMax=[]  SumI3OutMin=[]  SumI3OutMax=[]  SumI4OutMin=[]  SumI4OutMax=[]  SumDOutMin=[]  SumDOutMax=[]  DifferentiatorOutMin=[]  DifferentiatorOutMax=[]  FilterDiffOutCoefMin=[]  FilterDiffOutCoefMax=[]  ReciprocalOutMin=[]  ReciprocalOutMax=[]  SumDenOutMin=[]  SumDenOutMax=[]  SumNumOutMin=[]  SumNumOutMax=[]  DivideOutMin=[]  DivideOutMax=[]  UdiffTsProdOutMin=[]  UdiffTsProdOutMax=[]  NTsProdOutMin=[]  NTsProdOutMax=[]  UintegralTsProdOutMin=[]  UintegralTsProdOutMax=[]  UngainTsProdOutMin=[]  UngainTsProdOutMax=[]  ClampingZeroOutDataTypeStr=Inherit: Inherit via back propagation  ClampingZeroOutMin=[]  ClampingZeroOutMax=[]  FilterDenConstantOutDataTypeStr=Inherit: Inherit via back propagation  FilterDenConstantOutMin=[]  FilterDenConstantOutMax=[]  PCopyOutDataTypeStr=Inherit: Inherit via back propagation  PCopyOutMin=[]  PCopyOutMax=[]  NCopyOutDataTypeStr=Inherit: Inherit via back propagation  NCopyOutMin=[]  NCopyOutMax=[]  IntegratorContinuousStateAttributes=''  IntegratorStateMustResolveToSignalObject=off  IntegratorRTWStateStorageClass=Auto  FilterContinuousStateAttributes=''  FilterStateMustResolveToSignalObject=off  FilterRTWStateStorageClass=Auto  ParallelPVariant=InternalParameters  IdealPVariant=Disabled  IVariant=InternalParameters  DVariant=InternalParameters  IntegratorVariant=Discrete  SatVariant=Disabled  AWVariant=Passthrough  PCopyVariant=Disabled  TRVariant=Disabled  FdbkBlocksVariant=Forward  IdealPFdbkVariant=Disabled  SatFdbkVariant=Disabled  DerivativeFilterVariant=ForwardEulerFilter  NVariant=InternalParameters  NCopyVariant=Disabled  FilterICVariant=InternalICsFilter  IntegratorICVariant=InternalICs  ExternalResetVariant=Disabled  TRSumVariant=Passthrough  SumFdbkVariant=Disabled  SumVariant=Sum_PID  TsampFilterVariant=InternalTs  TsampNgainVariant=Passthrough  TsampIntegralVariant=Disabled_SignalSpec  ExternalSaturationOutDataTypeStr=Inherit: Same as second input
  PID Controller1 : slpidlib/PID Controller  Controller=PID  Form=Parallel  TimeDomain=Discrete-time  UseExternalTs=off  SampleTime=-1  IntegratorMethod=Forward Euler  FilterMethod=Forward Euler  ControllerParametersSource=internal  P=1.87988557248045  I=3  UseKiTs=off  D=0.151181707123562  N=252.206061331965  UseFilter=on  TunerSelectOption=Transfer Function Based (PID Tuner App)  InitialConditionSource=internal  InitialConditionForIntegrator=0  InitialConditionForFilter=0  DifferentiatorICPrevScaledInput=0  ExternalReset=none  TrackingMode=off  Kt=1  LimitOutput=off  SatLimitsSource=internal  UpperSaturationLimit=inf  LowerSaturationLimit=-inf  LinearizeAsGain=on  AntiWindupMode=none  Kb=1  LimitIntegrator=off  UpperIntegratorSaturationLimit=inf  LowerIntegratorSaturationLimit=-inf  POutMin=[]  POutMax=[]  IOutMin=[]  IOutMax=[]  DOutMin=[]  DOutMax=[]  NOutMin=[]  NOutMax=[]  SumOutMin=[]  SumOutMax=[]  SaturationOutMin=[]  SaturationOutMax=[]  PParamMin=[]  PParamMax=[]  IParamMin=[]  IParamMax=[]  DParamMin=[]  DParamMax=[]  NParamMin=[]  NParamMax=[]  KbParamMin=[]  KbParamMax=[]  KtParamMin=[]  KtParamMax=[]  KbOutMin=[]  KbOutMax=[]  KtOutMin=[]  KtOutMax=[]  IntegratorOutMin=[]  IntegratorOutMax=[]  FilterOutMin=[]  FilterOutMax=[]  SumI1OutMin=[]  SumI1OutMax=[]  SumI2OutMin=[]  SumI2OutMax=[]  SumI3OutMin=[]  SumI3OutMax=[]  SumI4OutMin=[]  SumI4OutMax=[]  SumDOutMin=[]  SumDOutMax=[]  DifferentiatorOutMin=[]  DifferentiatorOutMax=[]  FilterDiffOutCoefMin=[]  FilterDiffOutCoefMax=[]  ReciprocalOutMin=[]  ReciprocalOutMax=[]  SumDenOutMin=[]  SumDenOutMax=[]  SumNumOutMin=[]  SumNumOutMax=[]  DivideOutMin=[]  DivideOutMax=[]  UdiffTsProdOutMin=[]  UdiffTsProdOutMax=[]  NTsProdOutMin=[]  NTsProdOutMax=[]  UintegralTsProdOutMin=[]  UintegralTsProdOutMax=[]  UngainTsProdOutMin=[]  UngainTsProdOutMax=[]  ClampingZeroOutDataTypeStr=Inherit: Inherit via back propagation  ClampingZeroOutMin=[]  ClampingZeroOutMax=[]  FilterDenConstantOutDataTypeStr=Inherit: Inherit via back propagation  FilterDenConstantOutMin=[]  FilterDenConstantOutMax=[]  PCopyOutDataTypeStr=Inherit: Inherit via back propagation  PCopyOutMin=[]  PCopyOutMax=[]  NCopyOutDataTypeStr=Inherit: Inherit via back propagation  NCopyOutMin=[]  NCopyOutMax=[]  IntegratorContinuousStateAttributes=''  IntegratorStateMustResolveToSignalObject=off  IntegratorRTWStateStorageClass=Auto  FilterContinuousStateAttributes=''  FilterStateMustResolveToSignalObject=off  FilterRTWStateStorageClass=Auto  ParallelPVariant=InternalParameters  IdealPVariant=Disabled  IVariant=InternalParameters  DVariant=InternalParameters  IntegratorVariant=Discrete  SatVariant=Disabled  AWVariant=Passthrough  PCopyVariant=Disabled  TRVariant=Disabled  FdbkBlocksVariant=Forward  IdealPFdbkVariant=Disabled  SatFdbkVariant=Disabled  DerivativeFilterVariant=ForwardEulerFilter  NVariant=InternalParameters  NCopyVariant=Disabled  FilterICVariant=InternalICsFilter  IntegratorICVariant=InternalICs  ExternalResetVariant=Disabled  TRSumVariant=Passthrough  SumFdbkVariant=Disabled  SumVariant=Sum_PID  TsampFilterVariant=InternalTs  TsampNgainVariant=Passthrough  TsampIntegralVariant=Disabled_SignalSpec  ExternalSaturationOutDataTypeStr=Inherit: Same as second input
  Sum{,1..5} (6 alike) : Sum  Inputs=|+-
  cmd : Outport  VectorParamsAs1DForOutWhenUnconnected=off
  wires:
  Demux1/6 -> Sum5/2
  Demux1/5 -> Sum4/2
  Demux1/4 -> Sum3/2
  Demux1/3 -> Sum2/2
  Demux1/2 -> Sum1/2
  Demux/6 -> Sum5/1
  Demux/5 -> Sum4/1
  Demux/4 -> Sum3/1
  Demux/3 -> Sum2/1
  Demux/2 -> Sum1/1
  Mux/1 -> cmd/1
  Demux1/1 -> Sum/2
  Demux/1 -> Sum/1
  meas/1 -> Demux1/1
  ref/1 -> Demux/1
  Discrete PID Controller/1 -> Mux/1
  Discrete PID Controller2/1 -> Mux/3
  Discrete PID Controller3/1 -> Mux/4
  PID Controller1/1 -> Mux/5
  PID Controller/1 -> Mux/6
  Discrete PID Controller1/1 -> Mux/2
  Sum/1 -> Discrete PID Controller/1
  Sum1/1 -> Discrete PID Controller1/1
  Sum2/1 -> Discrete PID Controller2/1
  Sum3/1 -> Discrete PID Controller3/1
  Sum4/1 -> PID Controller1/1
  Sum5/1 -> PID Controller/1

== system TorqueControlConfig/Joint Controller (Configuration Space)/Saturate Inputs ==
  inp : Inport
  Saturate Joint Torques : Saturate  UpperLimit=200  LowerLimit=-200
  sat : Outport  VectorParamsAs1DForOutWhenUnconnected=off
  wires:
  Saturate Joint Torques/1 -> sat/1
  inp/1 -> Saturate Joint Torques/1

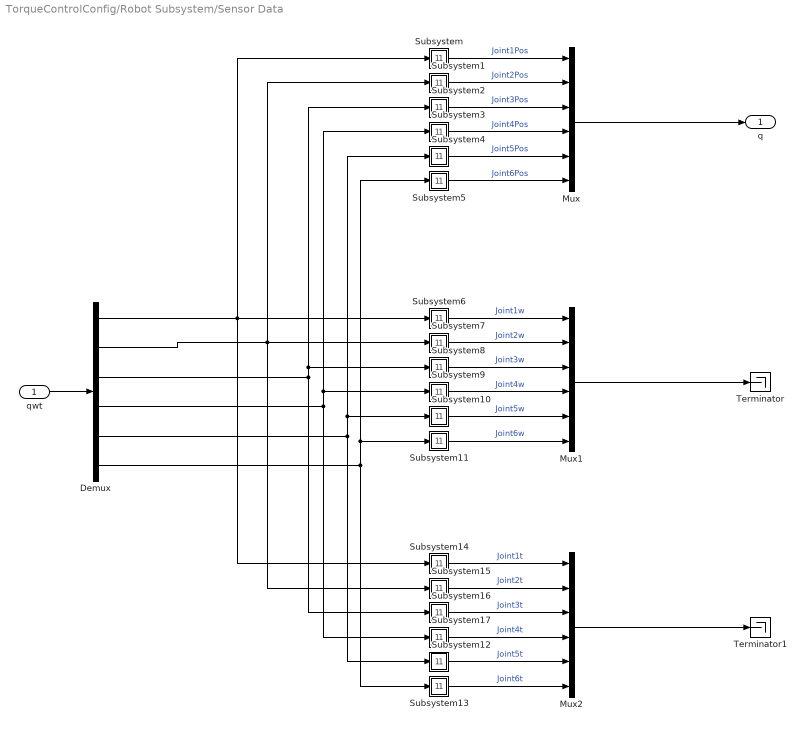
== system TorqueControlConfig/Robot Subsystem/Sensor Data ==
  qwt : Inport
  Demux : Demux  Outputs=6
  Mux : Mux  Inputs=6
  Mux1 : Mux  Inputs=6
  Mux2 : Mux  Inputs=6
  Subsystem : Subsystem
  Subsystem1 : Subsystem
  Subsystem10 : Subsystem
  Subsystem11 : Subsystem
  Subsystem12 : Subsystem
  Subsystem13 : Subsystem
  Subsystem14 : Subsystem
  Subsystem15 : Subsystem
  Subsystem16 : Subsystem
  Subsystem17 : Subsystem
  Subsystem2 : Subsystem
  Subsystem3 : Subsystem
  Subsystem4 : Subsystem
  Subsystem5 : Subsystem
  Subsystem6 : Subsystem
  Subsystem7 : Subsystem
  Subsystem8 : Subsystem
  Subsystem9 : Subsystem
  Terminator : Terminator
  Terminator1 : Terminator
  q : Outport
  wires:
  Subsystem1/1("  ") -> Mux/2  "Joint2Pos"
  Subsystem5/1("  ") -> Mux/6  "Joint6Pos"
  Subsystem/1("  ") -> Mux/1  "Joint1Pos"
  Subsystem3/1("  ") -> Mux/4  "Joint4Pos"
  Subsystem2/1("  ") -> Mux/3  "Joint3Pos"
  Subsystem4/1("  ") -> Mux/5  "Joint5Pos"
  Mux/1 -> q/1
  Subsystem7/1("  ") -> Mux1/2  "Joint2w"
  Subsystem6/1("  ") -> Mux1/1  "Joint1w"
  Subsystem9/1("  ") -> Mux1/4  "Joint4w"
  Subsystem11/1("  ") -> Mux1/6  "Joint6w"
  Subsystem8/1("  ") -> Mux1/3  "Joint3w"
  Mux1/1 -> Terminator/1
  Subsystem10/1("  ") -> Mux1/5  "Joint5w"
  Demux/5 -> Subsystem10/1(" "), Subsystem4/1(" "), Subsystem12/1(" ")
  Subsystem16/1("  ") -> Mux2/3  "Joint3t"
  Demux/4 -> Subsystem9/1(" "), Subsystem3/1(" "), Subsystem17/1(" ")
  Demux/2 -> Subsystem15/1(" "), Subsystem1/1(" "), Subsystem7/1(" ")
  Subsystem14/1("  ") -> Mux2/1  "Joint1t"
  Demux/6 -> Subsystem11/1(" "), Subsystem5/1(" "), Subsystem13/1(" ")
  Mux2/1 -> Terminator1/1
  Subsystem17/1("  ") -> Mux2/4  "Joint4t"
  Subsystem13/1("  ") -> Mux2/6  "Joint6t"
  Demux/1 -> Subsystem14/1(" "), Subsystem6/1(" "), Subsystem/1(" ")
  Subsystem15/1("  ") -> Mux2/2  "Joint2t"
  Demux/3 -> Subsystem8/1(" "), Subsystem2/1(" "), Subsystem16/1(" ")
  Subsystem12/1("  ") -> Mux2/5  "Joint5t"
  qwt/1 -> Demux/1

== system TorqueControlConfig/Robot Subsystem/tool0 ==
  ReferenceFrame : sm_lib/Frames and Transforms/Reference Frame
  F : PMIOPort  Side=Left
  connections:
  ReferenceFrame/RConn1 -- F/RConn1

== system TorqueControlConfig/CntrlManip/Switch1/Angle Value ==
  " " : Inport
  Constant : Constant  Value=0
  Constant1 : Constant  Value=0
  Simulink-PS Converter : nesl_utility/Simulink-PS Converter  PhysicalDomain=network_engine_domain  SubClassName=ps_input  LeftPortType=input  RightPortType=output  PseudoPeriodic=off  Frequencies=[]  NoiseDistribution=none  NoiseParameters=[]  Unit=rad  AffineConversion=off  FilteringAndDerivatives=provide  SimscapeFilterOrder=1  InputFilterTimeConstant=0.001  UdotUserProvided=2
  q : PMIOPort  Side=Right
  wires:
  " "/1 -> Simulink-PS Converter/1
  Constant/1 -> Simulink-PS Converter/2
  Constant1/1 -> Simulink-PS Converter/3
  connections:
  q/RConn1 -- Simulink-PS Converter/RConn1

== system TorqueControlConfig/CntrlManip/Switch2/Angle Value ==
  " " : Inport
  Constant : Constant  Value=0
  Constant1 : Constant  Value=0
  Simulink-PS Converter : nesl_utility/Simulink-PS Converter  PhysicalDomain=network_engine_domain  SubClassName=ps_input  LeftPortType=input  RightPortType=output  PseudoPeriodic=off  Frequencies=[]  NoiseDistribution=none  NoiseParameters=[]  Unit=rad  AffineConversion=off  FilteringAndDerivatives=provide  SimscapeFilterOrder=1  InputFilterTimeConstant=0.001  UdotUserProvided=2
  q : PMIOPort  Side=Right
  wires:
  " "/1 -> Simulink-PS Converter/1
  Constant/1 -> Simulink-PS Converter/2
  Constant1/1 -> Simulink-PS Converter/3
  connections:
  q/RConn1 -- Simulink-PS Converter/RConn1

== system TorqueControlConfig/CntrlManip/Switch3/Angle Value ==
  " " : Inport
  Constant : Constant  Value=0
  Constant1 : Constant  Value=0
  Simulink-PS Converter : nesl_utility/Simulink-PS Converter  PhysicalDomain=network_engine_domain  SubClassName=ps_input  LeftPortType=input  RightPortType=output  PseudoPeriodic=off  Frequencies=[]  NoiseDistribution=none  NoiseParameters=[]  Unit=rad  AffineConversion=off  FilteringAndDerivatives=provide  SimscapeFilterOrder=1  InputFilterTimeConstant=0.001  UdotUserProvided=2
  q : PMIOPort  Side=Right
  wires:
  " "/1 -> Simulink-PS Converter/1
  Constant/1 -> Simulink-PS Converter/2
  Constant1/1 -> Simulink-PS Converter/3
  connections:
  q/RConn1 -- Simulink-PS Converter/RConn1

== system TorqueControlConfig/CntrlManip/Switch4/Angle Value ==
  " " : Inport
  Constant : Constant  Value=0
  Constant1 : Constant  Value=0
  Simulink-PS Converter : nesl_utility/Simulink-PS Converter  PhysicalDomain=network_engine_domain  SubClassName=ps_input  LeftPortType=input  RightPortType=output  PseudoPeriodic=off  Frequencies=[]  NoiseDistribution=none  NoiseParameters=[]  Unit=rad  AffineConversion=off  FilteringAndDerivatives=provide  SimscapeFilterOrder=1  InputFilterTimeConstant=0.001  UdotUserProvided=2
  q : PMIOPort  Side=Right
  wires:
  " "/1 -> Simulink-PS Converter/1
  Constant/1 -> Simulink-PS Converter/2
  Constant1/1 -> Simulink-PS Converter/3
  connections:
  q/RConn1 -- Simulink-PS Converter/RConn1

== system TorqueControlConfig/CntrlManip/Switch5/Angle Value ==
  " " : Inport
  Constant : Constant  Value=0
  Constant1 : Constant  Value=0
  Simulink-PS Converter : nesl_utility/Simulink-PS Converter  PhysicalDomain=network_engine_domain  SubClassName=ps_input  LeftPortType=input  RightPortType=output  PseudoPeriodic=off  Frequencies=[]  NoiseDistribution=none  NoiseParameters=[]  Unit=rad  AffineConversion=off  FilteringAndDerivatives=provide  SimscapeFilterOrder=1  InputFilterTimeConstant=0.001  UdotUserProvided=2
  q : PMIOPort  Side=Right
  wires:
  " "/1 -> Simulink-PS Converter/1
  Constant/1 -> Simulink-PS Converter/2
  Constant1/1 -> Simulink-PS Converter/3
  connections:
  q/RConn1 -- Simulink-PS Converter/RConn1

== system TorqueControlConfig/CntrlManip/Switch6/Angle Value ==
  " " : Inport
  Constant : Constant  Value=0
  Constant1 : Constant  Value=0
  Simulink-PS Converter : nesl_utility/Simulink-PS Converter  PhysicalDomain=network_engine_domain  SubClassName=ps_input  LeftPortType=input  RightPortType=output  PseudoPeriodic=off  Frequencies=[]  NoiseDistribution=none  NoiseParameters=[]  Unit=rad  AffineConversion=off  FilteringAndDerivatives=provide  SimscapeFilterOrder=1  InputFilterTimeConstant=0.001  UdotUserProvided=2
  q : PMIOPort  Side=Right
  wires:
  " "/1 -> Simulink-PS Converter/1
  Constant/1 -> Simulink-PS Converter/2
  Constant1/1 -> Simulink-PS Converter/3
  connections:
  q/RConn1 -- Simulink-PS Converter/RConn1

== system TorqueControlConfig/Robot Subsystem/Sensor Data/Subsystem ==
  " " : Inport
  Demux1 : Demux  Outputs=3
  "  " : Outport
  wires:
  " "/1 -> Demux1/1
  Demux1/1 -> "  "/1

== system TorqueControlConfig/Robot Subsystem/Sensor Data/Subsystem1 ==
  " " : Inport
  Demux1 : Demux  Outputs=3
  "  " : Outport
  wires:
  Demux1/1 -> "  "/1
  " "/1 -> Demux1/1

== system TorqueControlConfig/Robot Subsystem/Sensor Data/Subsystem10 ==
  " " : Inport
  Demux1 : Demux  Outputs=3
  "  " : Outport
  wires:
  " "/1 -> Demux1/1
  Demux1/2 -> "  "/1

== system TorqueControlConfig/Robot Subsystem/Sensor Data/Subsystem11 ==
  " " : Inport
  Demux1 : Demux  Outputs=3
  "  " : Outport
  wires:
  Demux1/2 -> "  "/1
  " "/1 -> Demux1/1

== system TorqueControlConfig/Robot Subsystem/Sensor Data/Subsystem12 ==
  " " : Inport
  Demux1 : Demux  Outputs=3
  "  " : Outport
  wires:
  " "/1 -> Demux1/1
  Demux1/3 -> "  "/1

== system TorqueControlConfig/Robot Subsystem/Sensor Data/Subsystem13 ==
  " " : Inport
  Demux1 : Demux  Outputs=3
  "  " : Outport
  wires:
  Demux1/3 -> "  "/1
  " "/1 -> Demux1/1

== system TorqueControlConfig/Robot Subsystem/Sensor Data/Subsystem14 ==
  " " : Inport
  Demux1 : Demux  Outputs=3
  "  " : Outport
  wires:
  " "/1 -> Demux1/1
  Demux1/3 -> "  "/1
